simulink model "satellite_attitude_estimation_ekf_bst_model"  (R2017a)
settings: Solver=FixedStepAuto  StartTime=0.0  StopTime=10.0  FixedStep=dt  RelTol=1e-3
values from neighbouring files (symbols this model uses):
  ARW = N_ARW^2    (= 2.56183250041e-07)    [satellite_attitude_estimation_ekf_bst_run.m]
  dt = CONST.dt    [extended_kalman_filter.m]    (also in satellite_attitude_estimation_ekf_bst_run.m = 0.05)
  dt_mg = 1/20    (= 0.05)    [satellite_attitude_estimation_ekf_bst_run.m]
  dt_ss = 1/5    (= 0.2)    [satellite_attitude_estimation_ekf_bst_run.m]
  dt_st = 1    [satellite_attitude_estimation_ekf_bst_run.m]
  FOV = 70    [satellite_attitude_estimation_ekf_bst_run.m]
  Gg = eye(3).*(-0.01+0.02*rand(3))+              (ones(3,3)-eye(3)).*(-0.0006+0.0012*rand(3))    [satellite_attitude_estimation_ekf_bst_run.m]
  Gmg = eye(3).*(-0.02+0.04*rand(3)) +             (ones(3,3)-eye(3)).*(-0.0028+0.0056*rand(3))    [satellite_attitude_estimation_ekf_bst_run.m]
  GYRO_Bias = (3*randn(3,1))*pi/180    [satellite_attitude_estimation_ekf_bst_run.m]
  P = 2*pi*sqrt(a^3/CONST.mu)    [satellite_attitude_estimation_ekf_bst_run.m]
  q_B_I_0 = [q_I_B_0(1);-q_I_B_0(2);-q_I_B_0(3);-q_I_B_0(4)]    [satellite_attitude_estimation_ekf_bst_run.m]
  q_B_O_0 = [q_O_B_0(1);-q_O_B_0(2);-q_O_B_0(3);-q_O_B_0(4)]    [satellite_attitude_estimation_ekf_bst_run.m]
  R_S1_B = DCM(SSaxis(1),SSangles(1))    [satellite_attitude_estimation_ekf_bst_run.m]
  R_S2_B = DCM(SSaxis(2),SSangles(2))    [satellite_attitude_estimation_ekf_bst_run.m]
  R_S3_B = DCM(SSaxis(3),SSangles(3))    [satellite_attitude_estimation_ekf_bst_run.m]
  R_S4_B = DCM(SSaxis(4),SSangles(4))    [satellite_attitude_estimation_ekf_bst_run.m]
  RRW = K_RRW^2/3    (= 4.06156559716e-12)    [satellite_attitude_estimation_ekf_bst_run.m]
  sigMag = 1.25e-7    (= 1.25e-07)    [satellite_attitude_estimation_ekf_bst_run.m]
  sigSS = 0.1    [satellite_attitude_estimation_ekf_bst_run.m]
  varST = sigST^2    (= 1.27968566268e-08)    [satellite_attitude_estimation_ekf_bst_run.m]
  w_B_BI_0 = w_B_BO_0 + w_B_OI_0    [satellite_attitude_estimation_ekf_bst_run.m]
undefined symbols (not defined in the file or in its folder): R_0, V_0
libraries: simulink x5
settings Model: Creator=Rusty Goh  LastModifiedBy=Rusty Goh

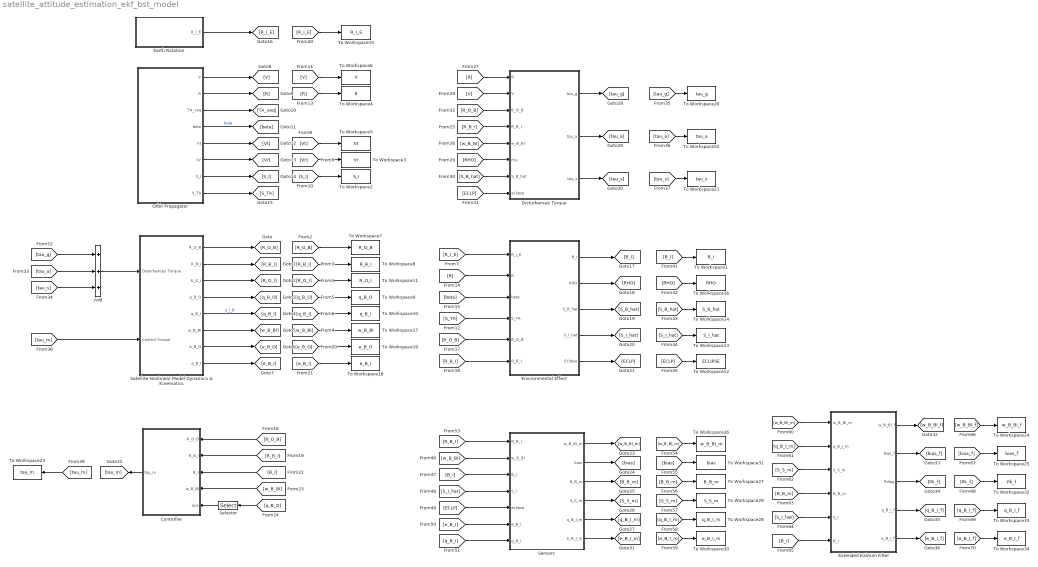
== system satellite_attitude_estimation_ekf_bst_model ==
  "\tOrbit Propagator" : Subsystem
  Add : Sum  Inputs=+++
  Controller : Subsystem
  Disturbances Torque : Subsystem
  Earth Rotation : Subsystem
  Environmental Effect : Subsystem
  Extended Kalman Filter : Subsystem
  Satellite Nonlinear Model Dynamics & Kinematics : Subsystem
  Selector : Selector  NumberOfDimensions=2  InputPortWidth=3  IndexOptions=Index vector (dialog),Index vector (dialog)  Indices=[2:4],1  OutputSizes=1,1
  Sensors : Subsystem
  To Workspace1 : ToWorkspace  VariableName=B_I  SampleTime=-1
  To Workspace10 : ToWorkspace  VariableName=q_B_I  SampleTime=-1
  To Workspace11 : ToWorkspace  VariableName=R_O_I  SampleTime=-1
  To Workspace12 : ToWorkspace  VariableName=ECLIPSE  SampleTime=-1
      settings: Save2DSignal=2-D array (concatenate along first dimension)
  To Workspace13 : ToWorkspace  VariableName=S_I_hat  SampleTime=-1
  To Workspace14 : ToWorkspace  VariableName=S_B_hat  SampleTime=-1
  To Workspace15 : ToWorkspace  VariableName=R_I_E  SampleTime=-1
  To Workspace16 : ToWorkspace  VariableName=RHO  SampleTime=-1
      settings: Save2DSignal=2-D array (concatenate along first dimension)
  To Workspace17 : ToWorkspace  VariableName=w_B_BI  SampleTime=-1
  To Workspace18 : ToWorkspace  VariableName=e_B_I  SampleTime=-1
  To Workspace19 : ToWorkspace  VariableName=e_B_O  SampleTime=-1
  To Workspace2 : ToWorkspace  VariableName=S_I  SampleTime=-1
  To Workspace20 : ToWorkspace  VariableName=tau_g  SampleTime=-1
  To Workspace21 : ToWorkspace  VariableName=tau_s  SampleTime=-1
  To Workspace22 : ToWorkspace  VariableName=tau_a  SampleTime=-1
      settings: Save2DSignal=2-D array (concatenate along first dimension)
  To Workspace23 : ToWorkspace  VariableName=tau_m  SampleTime=-1
  To Workspace24 : ToWorkspace  VariableName=w_B_BI_f  SampleTime=-1
  To Workspace25 : ToWorkspace  VariableName=bias_f  SampleTime=-1
  To Workspace26 : ToWorkspace  VariableName=w_B_BI_m  SampleTime=dt
  To Workspace27 : ToWorkspace  VariableName=B_B_m  SampleTime=dt
  To Workspace28 : ToWorkspace  VariableName=q_B_I_m  SampleTime=dt
  To Workspace29 : ToWorkspace  VariableName=S_S_m  SampleTime=dt
  To Workspace3 : ToWorkspace  VariableName=Vr  SampleTime=-1
  To Workspace30 : ToWorkspace  VariableName=e_B_I_m  SampleTime=dt
  To Workspace31 : ToWorkspace  VariableName=bias  SampleTime=dt
  To Workspace32 : ToWorkspace  VariableName=Pk_f  SampleTime=-1
  To Workspace33 : ToWorkspace  VariableName=q_B_I_f  SampleTime=-1
  To Workspace34 : ToWorkspace  VariableName=e_B_I_f  SampleTime=-1
  To Workspace4 : ToWorkspace  VariableName=R  SampleTime=-1
  To Workspace5 : ToWorkspace  VariableName=Vt  SampleTime=-1
  To Workspace6 : ToWorkspace  VariableName=V  SampleTime=-1
  To Workspace7 : ToWorkspace  VariableName=R_O_B  SampleTime=-1
  To Workspace8 : ToWorkspace  VariableName=R_B_I  SampleTime=-1
  To Workspace9 : ToWorkspace  VariableName=q_B_O  SampleTime=-1
  wires:
  Satellite Nonlinear Model Dynamics & Kinematics/4(q_B_O) -> [q_B_O]
  Satellite Nonlinear Model Dynamics & Kinematics/3(R_O_I) -> [R_O_I]
  Satellite Nonlinear Model Dynamics & Kinematics/1(R_O_B) -> [R_O_B]
  Satellite Nonlinear Model Dynamics & Kinematics/7(e_B_O) -> [e_B_O]
  Satellite Nonlinear Model Dynamics & Kinematics/5(q_B_I) -> [q_B_I]  "q_I_B"
  Satellite Nonlinear Model Dynamics & Kinematics/2(R_B_I) -> [R_B_I]
  Satellite Nonlinear Model Dynamics & Kinematics/6(w_B_BI) -> [w_B_BI]
  Satellite Nonlinear Model Dynamics & Kinematics/8(e_B_I) -> [e_B_I]
  Add/1 -> Satellite Nonlinear Model Dynamics & Kinematics/1(Disturbances Torque)
  "\tOrbit Propagator"/6(Vr) -> [Vr]
  "\tOrbit Propagator"/7("S_I ") -> [S_I]
  "\tOrbit Propagator"/3(TA_veq) -> [TA_veq]
  "\tOrbit Propagator"/4(beta) -> [beta]  "beta"
  "\tOrbit Propagator"/5(Vt) -> [Vt]
  "\tOrbit Propagator"/8(S_TA) -> [S_TA]
  "\tOrbit Propagator"/2(R) -> [R]
  "\tOrbit Propagator"/1(V) -> [V]
  [R] -> To Workspace4/1
  [Vr] -> To Workspace3/1
  [S_I] -> To Workspace2/1
  [Vt] -> To Workspace5/1
  [V] -> To Workspace6/1
  [R_O_B] -> To Workspace7/1
  [e_B_O] -> To Workspace19/1
  [w_B_BI] -> To Workspace17/1
  [R_O_I] -> To Workspace11/1
  [e_B_I] -> To Workspace18/1
  [R_B_I] -> To Workspace8/1
  [q_B_O] -> To Workspace9/1
  [q_B_I] -> To Workspace10/1
  [S_TA] -> Environmental Effect/4(S_TA)
  Environmental Effect/3(S_B_hat) -> [S_B_hat]
  [B_I] -> To Workspace1/1
  [ECLP] -> To Workspace12/1
  [R_I_E] -> To Workspace15/1
  [S_B_hat] -> To Workspace14/1
  [beta] -> Environmental Effect/3(beta)
  [R] -> Environmental Effect/2(R)
  Environmental Effect/5(Eclipse) -> [ECLP]
  [RHO] -> To Workspace16/1
  Environmental Effect/4(S_I_hat) -> [S_I_hat]
  Earth Rotation/1(R_I_E) -> [R_I_E]
  Environmental Effect/1(B_I) -> [B_I]
  Environmental Effect/2(RHO) -> [RHO]
  [S_I_hat] -> To Workspace13/1
  [R_B_I] -> Environmental Effect/6(R_B_I)
  [R_O_B] -> Environmental Effect/5(R_O_B)
  [R_I_E] -> Environmental Effect/1(R_I_E)
  Controller/1(tau_m) -> [tau_m]
  [R_O_B] -> Controller/1(R_O_B)
  [R_B_I] -> Controller/2(R_B_I)
  [B_I] -> Controller/3(B_I)
  [w_B_BI] -> Controller/4(w_B_BI)
  [q_B_O] -> Selector/1
  Selector/1 -> Controller/5(eps)
  [S_B_hat] -> Disturbances Torque/7(S_B_hat)
  [R_O_B] -> Disturbances Torque/3(R_O_B)
  [V] -> Disturbances Torque/2(V)
  Disturbances Torque/1(tau_g) -> [tau_g]
  [R_B_I] -> Disturbances Torque/4(R_B_I)
  [ECLP] -> Disturbances Torque/8(eclipse)
  [RHO] -> Disturbances Torque/6(rho)
  [w_B_BI] -> Disturbances Torque/5(w_B_BI)
  [R] -> Disturbances Torque/1(R)
  Disturbances Torque/2(tau_a) -> [tau_a]
  Disturbances Torque/3(tau_s) -> [tau_s]
  [tau_g] -> Add/1
  [tau_a] -> Add/2
  [tau_s] -> Add/3
  [tau_g] -> To Workspace20/1
  [tau_a] -> To Workspace22/1
  [tau_s] -> To Workspace21/1
  [tau_m] -> Satellite Nonlinear Model Dynamics & Kinematics/2(Control Torque)
  [tau_m] -> To Workspace23/1
  [S_S_m] -> To Workspace29/1
  [e_B_I_m] -> To Workspace30/1
  [B_B_m] -> To Workspace27/1
  [R_B_I] -> Sensors/1(R_B_I)
  [bias] -> To Workspace31/1
  [ECLP] -> Sensors/5(eclipse)
  [q_B_I] -> Sensors/7(q_B_I)
  [w_B_BI_m] -> To Workspace26/1
  [e_B_I] -> Sensors/6(e_B_I)
  Sensors/3(B_B_m) -> [B_B_m]
  Sensors/5(q_B_I_m) -> [q_B_I_m]
  [B_I] -> Sensors/3(B_I)
  Sensors/2(bias) -> [bias]
  Sensors/6(e_B_I_m) -> [e_B_I_m]
  [w_B_BI] -> Sensors/2(w_B_BI)
  [S_I_hat] -> Sensors/4(S_I)
  Sensors/4(S_S_m) -> [S_S_m]
  Sensors/1(w_B_BI_m) -> [w_B_BI_m]
  [q_B_I_m] -> To Workspace28/1
  [S_S_m] -> Extended Kalman Filter/3(S_S_m)
  Extended Kalman Filter/3(Pdiag) -> [Pk_f]
  Extended Kalman Filter/2(bias_f) -> [bias_f]
  [e_B_I_f] -> To Workspace34/1
  Extended Kalman Filter/4(q_B_I_f) -> [q_B_I_f]
  [Pk_f] -> To Workspace32/1
  [bias_f] -> To Workspace25/1
  [B_B_m] -> Extended Kalman Filter/4(B_B_m)
  [q_B_I_m] -> Extended Kalman Filter/2(q_B_I_m)
  Extended Kalman Filter/1(w_B_BI_f) -> [w_B_BI_f]
  [w_B_BI_f] -> To Workspace24/1
  [S_I_hat] -> Extended Kalman Filter/5(S_I)
  [q_B_I_f] -> To Workspace33/1
  [B_I] -> Extended Kalman Filter/6(B_I)
  Extended Kalman Filter/5(e_B_I_f) -> [e_B_I_f]
  [w_B_BI_m] -> Extended Kalman Filter/1(w_B_BI_m)

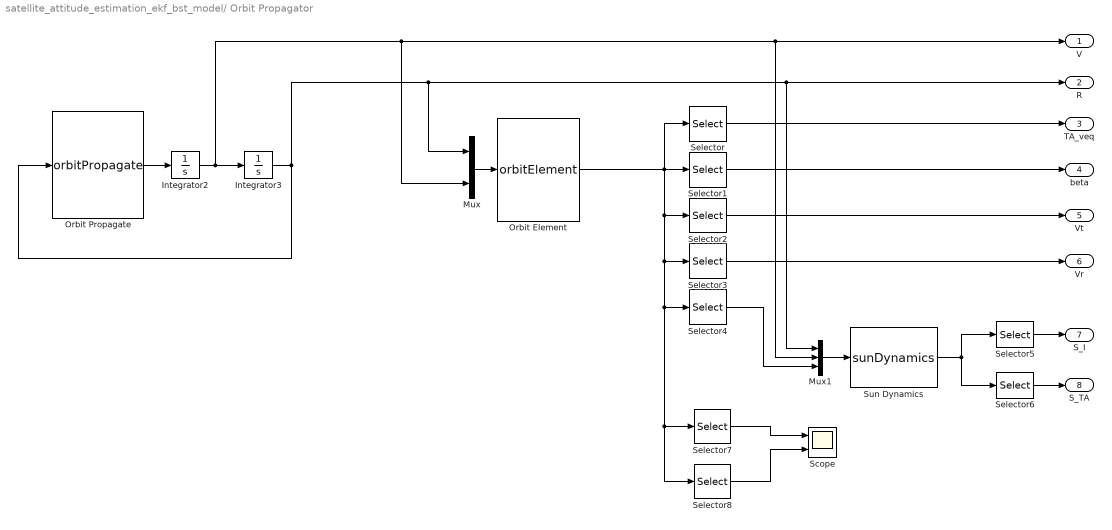
== system satellite_attitude_estimation_ekf_bst_model/	Orbit Propagator ==
  Integrator2 : Integrator  InitialCondition=V_0
  Integrator3 : Integrator  InitialCondition=R_0
  Mux : Mux  Inputs=2
  Mux1 : Mux  Inputs=3
  Orbit Element : MATLABFcn  MATLABFcn=orbitElement  OutputDimensions=11  Output1D=off
  Orbit Propagate : MATLABFcn  MATLABFcn=orbitPropagate  OutputDimensions=[3,1]  Output1D=off
  Scope : Scope  NumInputPorts=2
  Selector : Selector  InputPortWidth=11  IndexOptions=Index vector (dialog)  Indices=1  OutputSizes=1
  Selector1 : Selector  InputPortWidth=11  IndexOptions=Index vector (dialog)  Indices=2  OutputSizes=1
  Selector2 : Selector  InputPortWidth=11  IndexOptions=Index vector (dialog)  Indices=[3:5]  OutputSizes=1
  Selector3 : Selector  InputPortWidth=11  IndexOptions=Index vector (dialog)  Indices=[6:8]  OutputSizes=1
  Selector4 : Selector  InputPortWidth=11  IndexOptions=Index vector (dialog)  Indices=9  OutputSizes=1
  Selector5 : Selector  NumberOfDimensions=2  InputPortWidth=4  IndexOptions=Index vector (dialog),Index vector (dialog)  Indices=1:3,1  OutputSizes=1,1
  Selector6 : Selector  NumberOfDimensions=2  InputPortWidth=4  IndexOptions=Index vector (dialog),Index vector (dialog)  Indices=4,1  OutputSizes=1,1
  Selector7 : Selector  InputPortWidth=11  IndexOptions=Index vector (dialog)  Indices=10  OutputSizes=1
  Selector8 : Selector  InputPortWidth=11  IndexOptions=Index vector (dialog)  Indices=11  OutputSizes=1
  Sun Dynamics : MATLABFcn  MATLABFcn=sunDynamics  OutputDimensions=[4,1]  Output1D=off
  V : Outport
  R : Outport  Port=2
  TA_veq : Outport  Port=3
  beta : Outport  Port=4
  Vt : Outport  Port=5
  Vr : Outport  Port=6
  "S_I " : Outport  Port=7
  S_TA : Outport  Port=8
  wires:
  Mux/1 -> Orbit Element/1
  Orbit Element/1 -> Selector/1, Selector8/1, Selector7/1, Selector4/1, Selector3/1, Selector2/1, Selector1/1
  Orbit Propagate/1 -> Integrator2/1
  Integrator3/1 -> Mux/1, R/1, Mux1/1, Orbit Propagate/1
  Integrator2/1 -> Mux/2, Mux1/2, V/1, Integrator3/1
  Selector3/1 -> Vr/1
  Selector/1 -> TA_veq/1
  Selector2/1 -> Vt/1
  Selector1/1 -> beta/1
  Sun Dynamics/1 -> Selector6/1, Selector5/1
  Selector4/1 -> Mux1/3
  Selector6/1 -> S_TA/1
  Selector5/1 -> "S_I "/1
  Mux1/1 -> Sun Dynamics/1
  Selector7/1 -> Scope/1
  Selector8/1 -> Scope/2

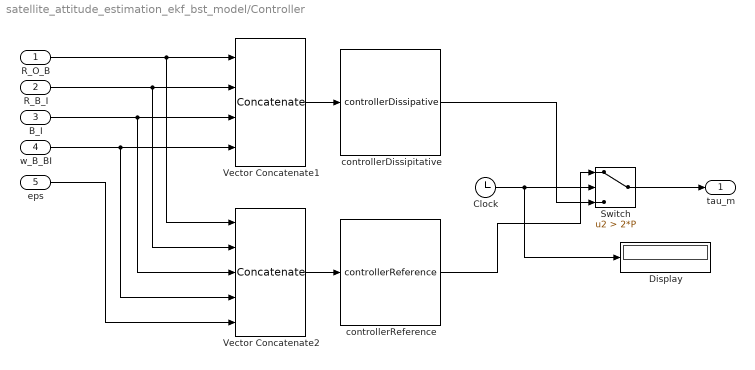
== system satellite_attitude_estimation_ekf_bst_model/Controller ==
  R_O_B : Inport
  R_B_I : Inport  Port=2
  B_I : Inport  Port=3
  w_B_BI : Inport  Port=4
  eps : Inport  Port=5
  Clock : Clock
  Display : Display
  Switch : Switch  Criteria=u2 > Threshold  Threshold=2*P
  Vector Concatenate1 : Concatenate  NumInputs=4  Mode=Multidimensional array  ConcatenateDimension=2
  Vector Concatenate2 : Concatenate  NumInputs=5  Mode=Multidimensional array  ConcatenateDimension=2
  controllerDissipitative : MATLABFcn  MATLABFcn=controllerDissipative  OutputDimensions=[3,1]  Output1D=off
  controllerReference : MATLABFcn  MATLABFcn=controllerReference  OutputDimensions=[3,1]  Output1D=off
  tau_m : Outport
  wires:
  Vector Concatenate1/1 -> controllerDissipitative/1
  R_O_B/1 -> Vector Concatenate2/1, Vector Concatenate1/1
  controllerDissipitative/1 -> Switch/3
  R_B_I/1 -> Vector Concatenate2/2, Vector Concatenate1/2
  B_I/1 -> Vector Concatenate2/3, Vector Concatenate1/3
  w_B_BI/1 -> Vector Concatenate2/4, Vector Concatenate1/4
  Vector Concatenate2/1 -> controllerReference/1
  eps/1 -> Vector Concatenate2/5
  controllerReference/1 -> Switch/1
  Clock/1 -> Display/1, Switch/2
  Switch/1 -> tau_m/1

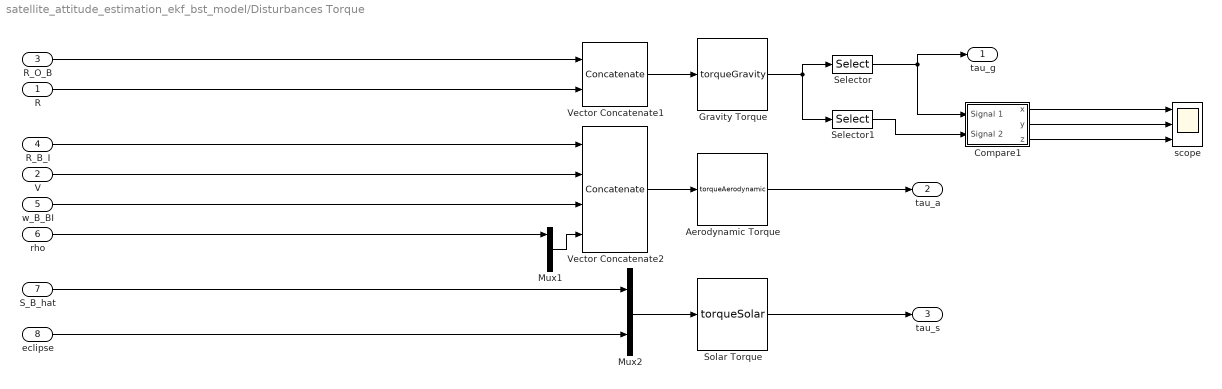
== system satellite_attitude_estimation_ekf_bst_model/Disturbances Torque ==
  R : Inport
  V : Inport  Port=2
  R_O_B : Inport  Port=3
  R_B_I : Inport  Port=4
  w_B_BI : Inport  Port=5
  rho : Inport  Port=6
  S_B_hat : Inport  Port=7
  eclipse : Inport  Port=8
  Aerodynamic Torque : MATLABFcn  MATLABFcn=torqueAerodynamic  OutputDimensions=[3,1]  Output1D=off
  Compare1 : Subsystem
  Gravity Torque : MATLABFcn  MATLABFcn=torqueGravity  OutputDimensions=[3,2]  Output1D=off
  Mux1 : Mux  Inputs=3
  Mux2 : Mux  Inputs=2
  Selector : Selector  NumberOfDimensions=2  InputPortWidth=3  IndexOptions=Index vector (dialog),Index vector (dialog)  Indices=[1:3],1  OutputSizes=1,1
  Selector1 : Selector  NumberOfDimensions=2  InputPortWidth=3  IndexOptions=Index vector (dialog),Index vector (dialog)  Indices=[1:3],2  OutputSizes=1,1
  Solar Torque : MATLABFcn  MATLABFcn=torqueSolar  OutputDimensions=[3,1]  Output1D=off
  Vector Concatenate1 : Concatenate  Mode=Multidimensional array  ConcatenateDimension=2
  Vector Concatenate2 : Concatenate  NumInputs=4  Mode=Multidimensional array  ConcatenateDimension=2
  scope : Scope  NumInputPorts=3
  tau_g : Outport
  tau_a : Outport  Port=2
  tau_s : Outport  Port=3
  wires:
  Vector Concatenate2/1 -> Aerodynamic Torque/1
  Mux1/1 -> Vector Concatenate2/4
  Vector Concatenate1/1 -> Gravity Torque/1
  Mux2/1 -> Solar Torque/1
  S_B_hat/1 -> Mux2/1
  w_B_BI/1 -> Vector Concatenate2/3
  R_B_I/1 -> Vector Concatenate2/1
  V/1 -> Vector Concatenate2/2
  R/1 -> Vector Concatenate1/2
  R_O_B/1 -> Vector Concatenate1/1
  rho/1 -> Mux1/1
  eclipse/1 -> Mux2/2
  Gravity Torque/1 -> Selector1/1, Selector/1
  Aerodynamic Torque/1 -> tau_a/1
  Solar Torque/1 -> tau_s/1
  Selector/1 -> tau_g/1, Compare1/1(Signal 1)
  Compare1/1(x) -> scope/1
  Compare1/2(y) -> scope/2
  Compare1/3(z) -> scope/3
  Selector1/1 -> Compare1/2(Signal 2)

== system satellite_attitude_estimation_ekf_bst_model/Earth Rotation ==
  Clock : Clock
  Interpreted MATLAB Function : MATLABFcn  MATLABFcn=earthDynamics  OutputDimensions=[3,3]  Output1D=off
  R_I_E : Outport
  wires:
  Interpreted MATLAB Function/1 -> R_I_E/1
  Clock/1 -> Interpreted MATLAB Function/1

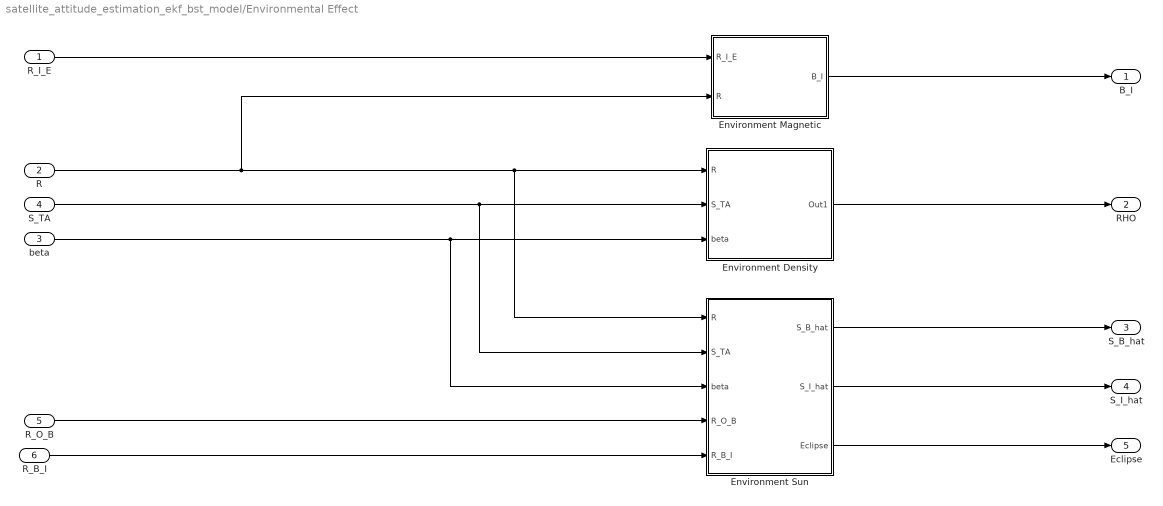
== system satellite_attitude_estimation_ekf_bst_model/Environmental Effect ==
  R_I_E : Inport
  R : Inport  Port=2
  beta : Inport  Port=3
  S_TA : Inport  Port=4
  R_O_B : Inport  Port=5
  R_B_I : Inport  Port=6
  Environment Density : Subsystem
  Environment Magnetic : Subsystem
  Environment Sun : Subsystem
  B_I : Outport
  RHO : Outport  Port=2
  S_B_hat : Outport  Port=3
  S_I_hat : Outport  Port=4
  Eclipse : Outport  Port=5
  wires:
  S_TA/1 -> Environment Sun/2(S_TA), Environment Density/2(S_TA)
  beta/1 -> Environment Sun/3(beta), Environment Density/3(beta)
  R_O_B/1 -> Environment Sun/4(R_O_B)
  R_B_I/1 -> Environment Sun/5(R_B_I)
  Environment Sun/1(S_B_hat) -> S_B_hat/1
  Environment Sun/2(S_I_hat) -> S_I_hat/1
  Environment Sun/3(Eclipse) -> Eclipse/1
  R/1 -> Environment Magnetic/2(R), Environment Sun/1(R), Environment Density/1(R)
  Environment Density/1(Out1) -> RHO/1
  R_I_E/1 -> Environment Magnetic/1(R_I_E)
  Environment Magnetic/1(B_I) -> B_I/1

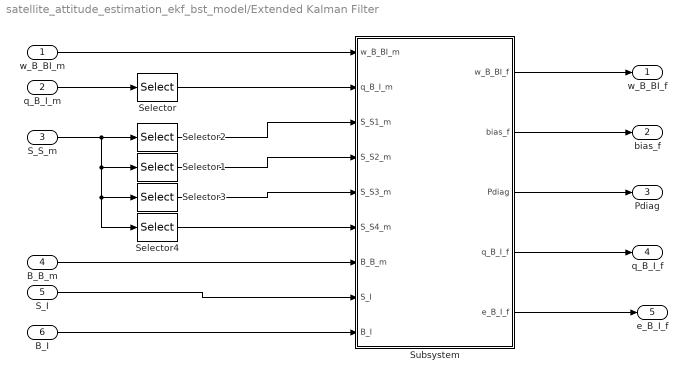
== system satellite_attitude_estimation_ekf_bst_model/Extended Kalman Filter ==
  w_B_BI_m : Inport
  q_B_I_m : Inport  Port=2
  S_S_m : Inport  Port=3
  B_B_m : Inport  Port=4
  S_I : Inport  Port=5
  B_I : Inport  Port=6
  Selector : Selector  InputPortWidth=4  IndexOptions=Index vector (dialog)  Indices=[2:4]  OutputSizes=1
  Selector1 : Selector  NumberOfDimensions=2  InputPortWidth=4  IndexOptions=Index vector (dialog),Index vector (dialog)  Indices=[1:3],2  OutputSizes=1,1
  Selector2 : Selector  NumberOfDimensions=2  InputPortWidth=4  IndexOptions=Index vector (dialog),Index vector (dialog)  Indices=[1:3],1  OutputSizes=1,1
  Selector3 : Selector  NumberOfDimensions=2  InputPortWidth=4  IndexOptions=Index vector (dialog),Index vector (dialog)  Indices=[1:3],3  OutputSizes=1,1
  Selector4 : Selector  NumberOfDimensions=2  InputPortWidth=4  IndexOptions=Index vector (dialog),Index vector (dialog)  Indices=[1:3],4  OutputSizes=1,1
  Subsystem : Subsystem
  w_B_BI_f : Outport
  bias_f : Outport  Port=2
  Pdiag : Outport  Port=3
  q_B_I_f : Outport  Port=4
  e_B_I_f : Outport  Port=5
  wires:
  q_B_I_m/1 -> Selector/1
  w_B_BI_m/1 -> Subsystem/1(w_B_BI_m)
  Selector2/1 -> Subsystem/3(S_S1_m)
  Selector1/1 -> Subsystem/4(S_S2_m)
  B_B_m/1 -> Subsystem/7(B_B_m)
  B_I/1 -> Subsystem/9(B_I)
  Selector/1 -> Subsystem/2(q_B_I_m)
  S_I/1 -> Subsystem/8(S_I)
  Subsystem/1(w_B_BI_f) -> w_B_BI_f/1
  Subsystem/2(bias_f) -> bias_f/1
  Subsystem/3(Pdiag) -> Pdiag/1
  Subsystem/4(q_B_I_f) -> q_B_I_f/1
  Subsystem/5(e_B_I_f) -> e_B_I_f/1
  S_S_m/1 -> Selector2/1, Selector4/1, Selector3/1, Selector1/1
  Selector3/1 -> Subsystem/5(S_S3_m)
  Selector4/1 -> Subsystem/6(S_S4_m)

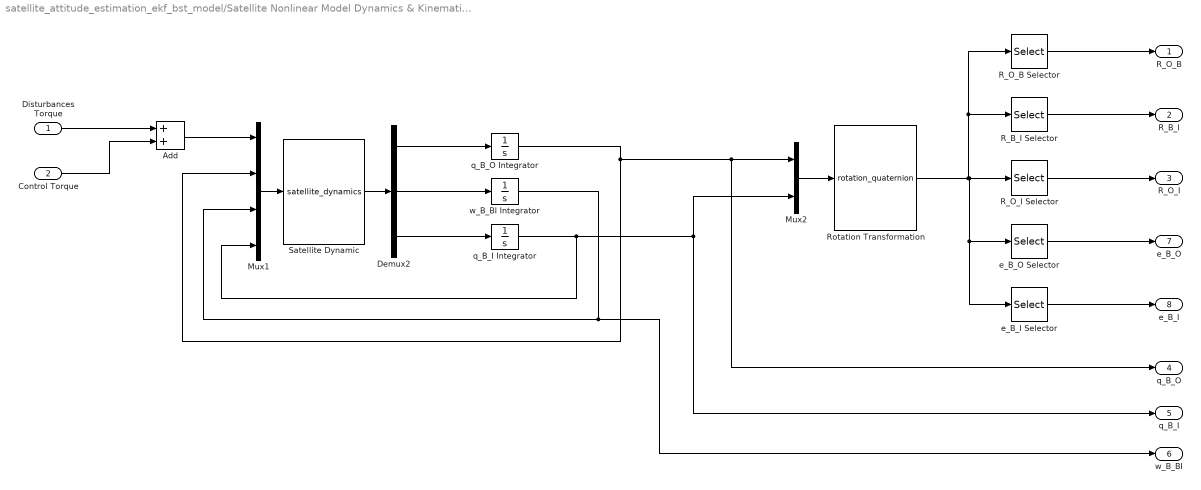
== system satellite_attitude_estimation_ekf_bst_model/Satellite Nonlinear Model Dynamics & Kinematics ==
  Disturbances Torque : Inport
  Control Torque : Inport  Port=2
  " w_B_BI Integrator" : Integrator  InitialCondition=w_B_BI_0
  Add : Sum
  Demux2 : Demux  Outputs=[4 3 4]
  Mux1 : Mux  Inputs=[3 4 3 4]
  Mux2 : Mux  Inputs=[4 4]
  R_B_I Selector : Selector  NumberOfDimensions=2  InputPortWidth=3  IndexOptions=Index vector (dialog),Index vector (dialog)  Indices=[1:3],[4:6]  OutputSizes=1,1
  R_O_B Selector : Selector  NumberOfDimensions=2  InputPortWidth=3  IndexOptions=Index vector (dialog),Index vector (dialog)  Indices=[1:3],[1:3]  OutputSizes=1,1
  R_O_I Selector : Selector  NumberOfDimensions=2  InputPortWidth=3  IndexOptions=Index vector (dialog),Index vector (dialog)  Indices=[1:3],[7:9]  OutputSizes=1,1
  Rotation Transformation : MATLABFcn  MATLABFcn=rotation_quaternion  OutputDimensions=[3,11]  Output1D=off
  Satellite Dynamic : MATLABFcn  MATLABFcn=satellite_dynamics  OutputDimensions=[11,1]  Output1D=off
  e_B_I Selector : Selector  NumberOfDimensions=2  InputPortWidth=3  IndexOptions=Index vector (dialog),Index vector (dialog)  Indices=[1:3],11  OutputSizes=1,1
  e_B_O Selector : Selector  NumberOfDimensions=2  InputPortWidth=3  IndexOptions=Index vector (dialog),Index vector (dialog)  Indices=[1:3],10  OutputSizes=1,1
  q_B_I Integrator : Integrator  InitialCondition=q_B_I_0
  q_B_O Integrator : Integrator  InitialCondition=q_B_O_0
  R_O_B : Outport
  R_B_I : Outport  Port=2
  R_O_I : Outport  Port=3
  q_B_O : Outport  Port=4
  q_B_I : Outport  Port=5
  w_B_BI : Outport  Port=6
  e_B_O : Outport  Port=7
  e_B_I : Outport  Port=8
  wires:
  R_O_I Selector/1 -> R_O_I/1
  q_B_O Integrator/1 -> Mux2/1, q_B_O/1, Mux1/2
  Satellite Dynamic/1 -> Demux2/1
  Disturbances Torque/1 -> Add/1
  Demux2/2 -> " w_B_BI Integrator"/1
  Demux2/3 -> q_B_I Integrator/1
  q_B_I Integrator/1 -> Mux2/2, q_B_I/1, Mux1/4
  Mux1/1 -> Satellite Dynamic/1
  Rotation Transformation/1 -> R_O_B Selector/1, R_B_I Selector/1, e_B_I Selector/1, e_B_O Selector/1, R_O_I Selector/1
  " w_B_BI Integrator"/1 -> w_B_BI/1, Mux1/3
  Demux2/1 -> q_B_O Integrator/1
  Mux2/1 -> Rotation Transformation/1
  R_B_I Selector/1 -> R_B_I/1
  R_O_B Selector/1 -> R_O_B/1
  Control Torque/1 -> Add/2
  Add/1 -> Mux1/1
  e_B_I Selector/1 -> e_B_I/1
  e_B_O Selector/1 -> e_B_O/1

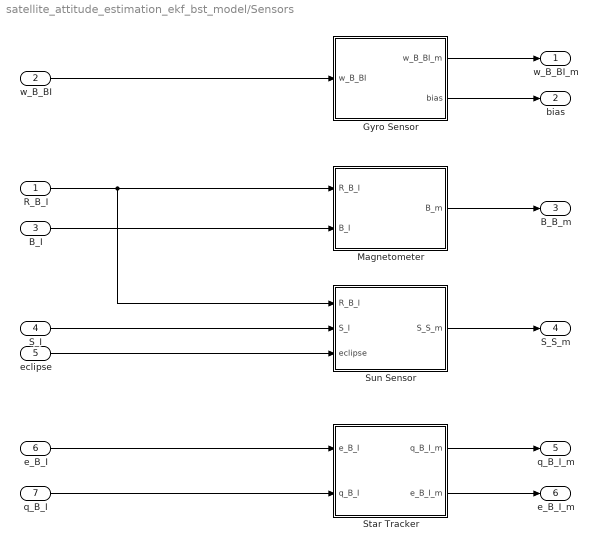
== system satellite_attitude_estimation_ekf_bst_model/Sensors ==
  R_B_I : Inport
  w_B_BI : Inport  Port=2
  B_I : Inport  Port=3
  S_I : Inport  Port=4
  eclipse : Inport  Port=5
  e_B_I : Inport  Port=6
  q_B_I : Inport  Port=7
  Gyro Sensor : Subsystem
  Magnetometer : Subsystem
  Star Tracker : Subsystem
  Sun Sensor : Subsystem
  w_B_BI_m : Outport
  bias : Outport  Port=2
  B_B_m : Outport  Port=3
  S_S_m : Outport  Port=4
  q_B_I_m : Outport  Port=5
  e_B_I_m : Outport  Port=6
  wires:
  e_B_I/1 -> Star Tracker/1(e_B_I)
  B_I/1 -> Magnetometer/2(B_I)
  eclipse/1 -> Sun Sensor/3(eclipse)
  Sun Sensor/1(S_S_m) -> S_S_m/1
  Gyro Sensor/2(bias) -> bias/1
  Gyro Sensor/1(w_B_BI_m) -> w_B_BI_m/1
  Star Tracker/1(q_B_I_m) -> q_B_I_m/1
  Magnetometer/1(B_m) -> B_B_m/1
  w_B_BI/1 -> Gyro Sensor/1(w_B_BI)
  S_I/1 -> Sun Sensor/2(S_I)
  R_B_I/1 -> Sun Sensor/1(R_B_I), Magnetometer/1(R_B_I)
  q_B_I/1 -> Star Tracker/2(q_B_I)
  Star Tracker/2(e_B_I_m) -> e_B_I_m/1

== system satellite_attitude_estimation_ekf_bst_model/Disturbances Torque/Compare1 ==
  Signal 1 : Inport
  Signal 2 : Inport  Port=2
  Demux3 : Demux  Outputs=3
  Demux4 : Demux  Outputs=3
  Mux : Mux  Inputs=2
  Mux1 : Mux  Inputs=2
  Mux2 : Mux  Inputs=2
  x : Outport
  y : Outport  Port=2
  z : Outport  Port=3
  wires:
  Demux3/3 -> Mux2/2
  Demux3/2 -> Mux1/2
  Demux4/2 -> Mux1/1
  Demux3/1 -> Mux/2
  Mux/1 -> x/1
  Mux2/1 -> z/1
  Demux4/1 -> Mux/1
  Mux1/1 -> y/1
  Demux4/3 -> Mux2/1
  Signal 2/1 -> Demux3/1
  Signal 1/1 -> Demux4/1

== system satellite_attitude_estimation_ekf_bst_model/Environmental Effect/Environment Density ==
  R : Inport
  S_TA : Inport  Port=2
  beta : Inport  Port=3
  Environment Density : MATLABFcn  MATLABFcn=environmentDensity  OutputDimensions=1  Output1D=off
  Mux : Mux  Inputs=3
  Out1 : Outport
  wires:
  Mux/1 -> Environment Density/1
  Environment Density/1 -> Out1/1
  S_TA/1 -> Mux/2
  beta/1 -> Mux/3
  R/1 -> Mux/1

== system satellite_attitude_estimation_ekf_bst_model/Environmental Effect/Environment Magnetic ==
  R_I_E : Inport
  R : Inport  Port=2
  Environment Magnetic : MATLABFcn  MATLABFcn=environmentMagnetic  OutputDimensions=[3,1]  Output1D=off
  Vector Concatenate : Concatenate  Mode=Multidimensional array  ConcatenateDimension=2
  B_I : Outport
  wires:
  R_I_E/1 -> Vector Concatenate/1
  Vector Concatenate/1 -> Environment Magnetic/1
  R/1 -> Vector Concatenate/2
  Environment Magnetic/1 -> B_I/1

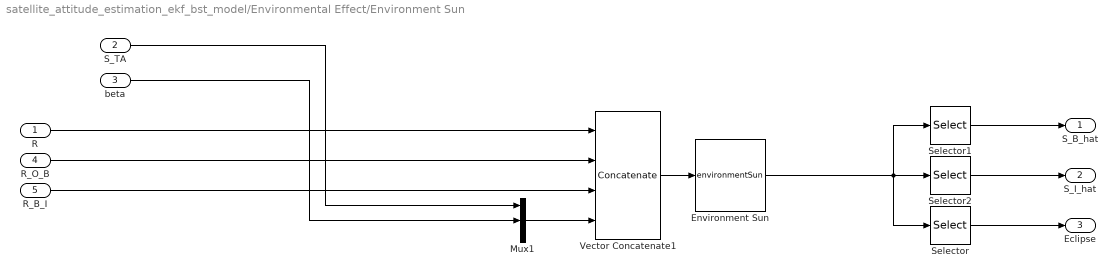
== system satellite_attitude_estimation_ekf_bst_model/Environmental Effect/Environment Sun ==
  R : Inport
  S_TA : Inport  Port=2
  beta : Inport  Port=3
  R_O_B : Inport  Port=4
  R_B_I : Inport  Port=5
  Environment Sun : MATLABFcn  MATLABFcn=environmentSun  OutputDimensions=[3,3]  Output1D=off
  Mux1 : Mux  Inputs=3
  Selector : Selector  NumberOfDimensions=2  InputPortWidth=3  IndexOptions=Index vector (dialog),Index vector (dialog)  Indices=3,3  OutputSizes=1,1
  Selector1 : Selector  NumberOfDimensions=2  InputPortWidth=3  IndexOptions=Index vector (dialog),Index vector (dialog)  Indices=[1:3],1  OutputSizes=1,1
  Selector2 : Selector  NumberOfDimensions=2  InputPortWidth=3  IndexOptions=Index vector (dialog),Index vector (dialog)  Indices=[1:3],2  OutputSizes=1,1
  Vector Concatenate1 : Concatenate  NumInputs=4  Mode=Multidimensional array  ConcatenateDimension=2
  S_B_hat : Outport
  S_I_hat : Outport  Port=2
  Eclipse : Outport  Port=3
  wires:
  R/1 -> Vector Concatenate1/1
  Mux1/1 -> Vector Concatenate1/4
  Selector/1 -> Eclipse/1
  Selector1/1 -> S_B_hat/1
  Vector Concatenate1/1 -> Environment Sun/1
  R_O_B/1 -> Vector Concatenate1/2
  R_B_I/1 -> Vector Concatenate1/3
  Selector2/1 -> S_I_hat/1
  Environment Sun/1 -> Selector/1, Selector1/1, Selector2/1
  S_TA/1 -> Mux1/1
  beta/1 -> Mux1/2

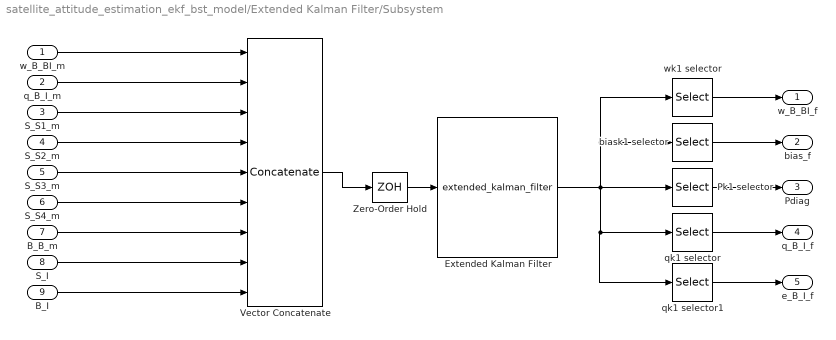
== system satellite_attitude_estimation_ekf_bst_model/Extended Kalman Filter/Subsystem ==
  w_B_BI_m : Inport
  q_B_I_m : Inport  Port=2
  S_S1_m : Inport  Port=3
  S_S2_m : Inport  Port=4
  S_S3_m : Inport  Port=5
  S_S4_m : Inport  Port=6
  B_B_m : Inport  Port=7
  S_I : Inport  Port=8
  B_I : Inport  Port=9
  Extended Kalman Filter : MATLABFcn  MATLABFcn=extended_kalman_filter  OutputDimensions=[6,9]  Output1D=off
  Pk1 selector : Selector  NumberOfDimensions=2  InputPortWidth=3  IndexOptions=Index vector (dialog),Index vector (dialog)  Indices=[1:6],[2:7]  OutputSizes=1,1
  Vector Concatenate : Concatenate  NumInputs=9  Mode=Multidimensional array  ConcatenateDimension=2
  Zero-Order Hold : ZeroOrderHold  SampleTime=dt
  biask1 selector : Selector  NumberOfDimensions=2  InputPortWidth=3  IndexOptions=Index vector (dialog),Index vector (dialog)  Indices=[4:6],1  OutputSizes=1,1
  qk1 selector : Selector  NumberOfDimensions=2  InputPortWidth=3  IndexOptions=Index vector (dialog),Index vector (dialog)  Indices=[1:4],8  OutputSizes=1,1
  qk1 selector1 : Selector  NumberOfDimensions=2  InputPortWidth=3  IndexOptions=Index vector (dialog),Index vector (dialog)  Indices=[1:3],9  OutputSizes=1,1
  wk1 selector : Selector  NumberOfDimensions=2  InputPortWidth=3  IndexOptions=Index vector (dialog),Index vector (dialog)  Indices=[1:3],1  OutputSizes=1,1
  w_B_BI_f : Outport
  bias_f : Outport  Port=2
  Pdiag : Outport  Port=3
  q_B_I_f : Outport  Port=4
  e_B_I_f : Outport  Port=5
  wires:
  Vector Concatenate/1 -> Zero-Order Hold/1
  S_S2_m/1 -> Vector Concatenate/4
  Pk1 selector/1 -> Pdiag/1
  qk1 selector1/1 -> e_B_I_f/1
  qk1 selector/1 -> q_B_I_f/1
  B_B_m/1 -> Vector Concatenate/7
  S_S1_m/1 -> Vector Concatenate/3
  Extended Kalman Filter/1 -> wk1 selector/1, biask1 selector/1, qk1 selector1/1, qk1 selector/1, Pk1 selector/1
  S_I/1 -> Vector Concatenate/8
  q_B_I_m/1 -> Vector Concatenate/2
  wk1 selector/1 -> w_B_BI_f/1
  w_B_BI_m/1 -> Vector Concatenate/1
  B_I/1 -> Vector Concatenate/9
  biask1 selector/1 -> bias_f/1
  Zero-Order Hold/1 -> Extended Kalman Filter/1
  S_S3_m/1 -> Vector Concatenate/5
  S_S4_m/1 -> Vector Concatenate/6

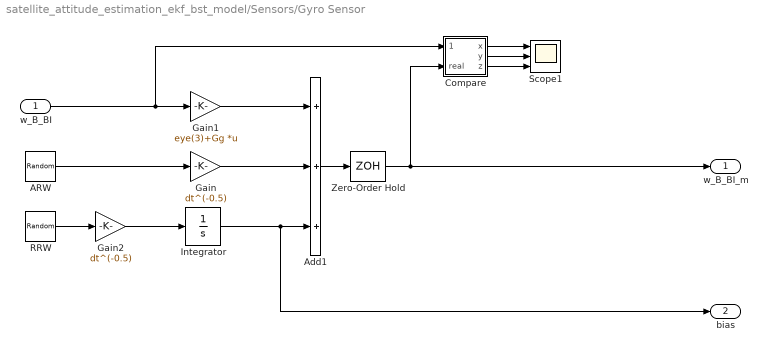
== system satellite_attitude_estimation_ekf_bst_model/Sensors/Gyro Sensor ==
  w_B_BI : Inport
  ARW : RandomNumber  Variance=[ARW;ARW;ARW]  SampleTime=dt  VectorParams1D=off
  Add1 : Sum  Inputs=+++
  Compare : Subsystem
  Gain : Gain  Gain=dt^(-0.5)
  Gain1 : Gain  Gain=eye(3)+Gg  Multiplication=Matrix(K*u)
  Gain2 : Gain  Gain=dt^(-0.5)
  Integrator : Integrator  InitialCondition=GYRO_Bias
  RRW : RandomNumber  Variance=[RRW;RRW;RRW]  SampleTime=dt  VectorParams1D=off
  Scope1 : Scope  NumInputPorts=3
  Zero-Order Hold : ZeroOrderHold  SampleTime=dt
  w_B_BI_m : Outport
  bias : Outport  Port=2
  wires:
  w_B_BI/1 -> Compare/1(true), Gain1/1
  Gain/1 -> Add1/2
  ARW/1 -> Gain/1
  Add1/1 -> Zero-Order Hold/1
  RRW/1 -> Gain2/1
  Integrator/1 -> Add1/3, bias/1
  Gain1/1 -> Add1/1
  Zero-Order Hold/1 -> w_B_BI_m/1, Compare/2(real)
  Compare/2(y) -> Scope1/2
  Compare/3(z) -> Scope1/3
  Compare/1(x) -> Scope1/1
  Gain2/1 -> Integrator/1

== system satellite_attitude_estimation_ekf_bst_model/Sensors/Magnetometer ==
  R_B_I : Inport
  B_I : Inport  Port=2
  ARW : RandomNumber  Variance=[sigMag^2;sigMag^2;sigMag^2]  SampleTime=dt_mg  VectorParams1D=off
  Add1 : Sum
  Compare : Subsystem
  Matrix Multiply : Product  Multiplication=Matrix(*)
  ScaleFactor MissAlignment : Gain  Gain=eye(3) + Gmg  Multiplication=Matrix(K*u)
  Scope1 : Scope  NumInputPorts=3
  Zero-Order Hold : ZeroOrderHold  SampleTime=dt_mg
  B_m : Outport
  wires:
  Matrix Multiply/1 -> Compare/1(true), ScaleFactor MissAlignment/1  "B_B"
  ScaleFactor MissAlignment/1 -> Add1/1
  Add1/1 -> Zero-Order Hold/1
  ARW/1 -> Add1/2
  B_I/1 -> Matrix Multiply/2
  R_B_I/1 -> Matrix Multiply/1
  Compare/2(y) -> Scope1/2
  Compare/3(z) -> Scope1/3
  Compare/1(x) -> Scope1/1
  Zero-Order Hold/1 -> Compare/2(real), B_m/1

== system satellite_attitude_estimation_ekf_bst_model/Sensors/Star Tracker ==
  e_B_I : Inport
  q_B_I : Inport  Port=2
  Mux : Mux  Inputs=2
  ST Noise : RandomNumber  Variance=[varST;varST;varST]  SampleTime=dt_st  VectorParams1D=off
  Selector : Selector  InputPortWidth=8  IndexOptions=Index vector (dialog)  Indices=[1:4]  OutputSizes=1
  Star Tracker : MATLABFcn  MATLABFcn=sensor_startracker  OutputDimensions=[8,1]  Output1D=off
  Sum : Sum  Inputs=|++
  Zero-Order Hold : ZeroOrderHold  SampleTime=dt_st
  q_B_I_m : Outport
  e_B_I_m : Outport  Port=2
  wires:
  Mux/1 -> Star Tracker/1
  Selector/1 -> Zero-Order Hold/1
  ST Noise/1 -> Sum/2
  e_B_I/1 -> Sum/1
  Star Tracker/1 -> Selector/1
  Zero-Order Hold/1 -> q_B_I_m/1
  Sum/1 -> e_B_I_m/1, Mux/2
  q_B_I/1 -> Mux/1

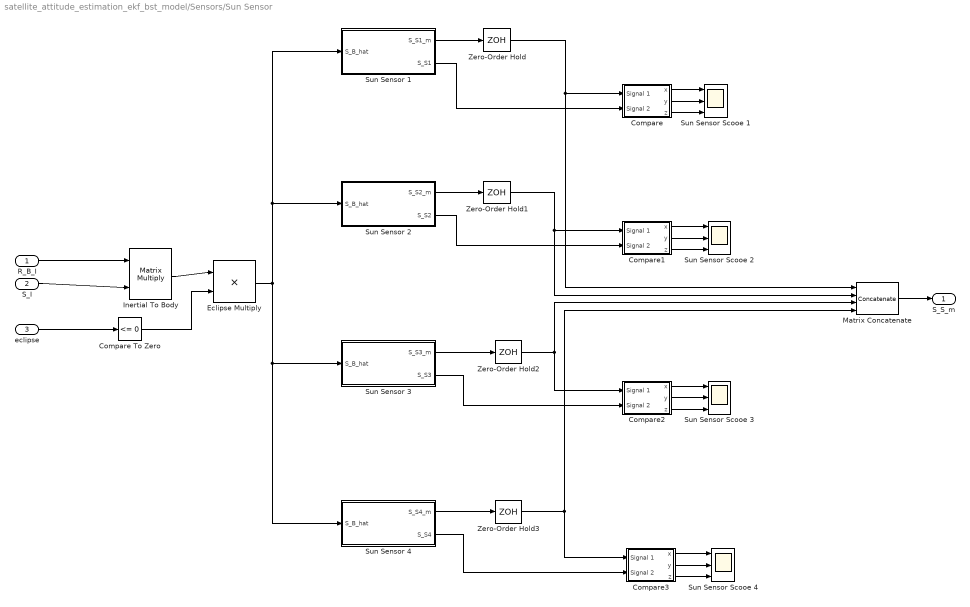
== system satellite_attitude_estimation_ekf_bst_model/Sensors/Sun Sensor ==
  R_B_I : Inport
  S_I : Inport  Port=2
  eclipse : Inport  Port=3
  Compare : Subsystem
  Compare To Zero : simulink/Logic and Bit Operations/Compare To Zero  relop=<=  OutDataTypeStr=boolean
  Compare1 : Subsystem
  Compare2 : Subsystem
  Compare3 : Subsystem
  Eclipse Multiply : Product
  Inertial To Body : Product  Multiplication=Matrix(*)
  Matrix Concatenate : Concatenate  NumInputs=4  Mode=Multidimensional array  ConcatenateDimension=2
  Sun Sensor Scooe {1..4} (4 alike) : Scope  NumInputPorts=3
  Sun Sensor 1 : Subsystem
  Sun Sensor 2 : Subsystem
  Sun Sensor 3 : Subsystem
  Sun Sensor 4 : Subsystem
  Zero-Order Hold{,1..3} (4 alike) : ZeroOrderHold  SampleTime=dt_ss
  S_S_m : Outport
  wires:
  R_B_I/1 -> Inertial To Body/1
  S_I/1 -> Inertial To Body/2
  Eclipse Multiply/1 -> Sun Sensor 1/1(S_B_hat), Sun Sensor 2/1(S_B_hat), Sun Sensor 4/1(S_B_hat), Sun Sensor 3/1(S_B_hat)
  Matrix Concatenate/1 -> S_S_m/1
  Inertial To Body/1 -> Eclipse Multiply/1
  Compare To Zero/1 -> Eclipse Multiply/2
  eclipse/1 -> Compare To Zero/1
  Sun Sensor 1/1(S_S1_m) -> Zero-Order Hold/1
  Sun Sensor 2/1(S_S2_m) -> Zero-Order Hold1/1
  Zero-Order Hold/1 -> Compare/1(Signal 1), Matrix Concatenate/1
  Zero-Order Hold1/1 -> Compare1/1(Signal 1), Matrix Concatenate/2
  Sun Sensor 1/2(S_S1) -> Compare/2(Signal 2)
  Compare/1(x) -> Sun Sensor Scooe 1/1
  Compare/2(y) -> Sun Sensor Scooe 1/2
  Compare/3(z) -> Sun Sensor Scooe 1/3
  Sun Sensor 3/1(S_S3_m) -> Zero-Order Hold2/1
  Sun Sensor 4/1(S_S4_m) -> Zero-Order Hold3/1
  Zero-Order Hold2/1 -> Compare2/1(Signal 1), Matrix Concatenate/3
  Zero-Order Hold3/1 -> Compare3/1(Signal 1), Matrix Concatenate/4
  Compare1/2(y) -> Sun Sensor Scooe 2/2
  Compare1/1(x) -> Sun Sensor Scooe 2/1
  Compare1/3(z) -> Sun Sensor Scooe 2/3
  Sun Sensor 2/2(S_S2) -> Compare1/2(Signal 2)
  Compare2/2(y) -> Sun Sensor Scooe 3/2
  Compare2/1(x) -> Sun Sensor Scooe 3/1
  Compare2/3(z) -> Sun Sensor Scooe 3/3
  Sun Sensor 3/2(S_S3) -> Compare2/2(Signal 2)
  Compare3/2(y) -> Sun Sensor Scooe 4/2
  Compare3/1(x) -> Sun Sensor Scooe 4/1
  Compare3/3(z) -> Sun Sensor Scooe 4/3
  Sun Sensor 4/2(S_S4) -> Compare3/2(Signal 2)

== system satellite_attitude_estimation_ekf_bst_model/Sensors/Gyro Sensor/Compare ==
  true : Inport
  real : Inport  Port=2
  Demux : Demux  Outputs=3
  Demux1 : Demux  Outputs=3
  Mux : Mux  Inputs=2
  Mux1 : Mux  Inputs=2
  Mux2 : Mux  Inputs=2
  x : Outport
  y : Outport  Port=2
  z : Outport  Port=3
  wires:
  Mux1/1 -> y/1
  Mux2/1 -> z/1
  true/1 -> Demux/1
  real/1 -> Demux1/1
  Mux/1 -> x/1
  Demux1/3 -> Mux2/2
  Demux1/2 -> Mux1/2
  Demux/3 -> Mux2/1
  Demux/1 -> Mux/1
  Demux/2 -> Mux1/1
  Demux1/1 -> Mux/2

== system satellite_attitude_estimation_ekf_bst_model/Sensors/Magnetometer/Compare ==
  true : Inport
  real : Inport  Port=2
  Demux : Demux  Outputs=3
  Demux1 : Demux  Outputs=3
  Mux : Mux  Inputs=2
  Mux1 : Mux  Inputs=2
  Mux2 : Mux  Inputs=2
  x : Outport
  y : Outport  Port=2
  z : Outport  Port=3
  wires:
  Mux1/1 -> y/1
  Mux2/1 -> z/1
  true/1 -> Demux/1
  real/1 -> Demux1/1
  Mux/1 -> x/1
  Demux1/3 -> Mux2/2
  Demux1/2 -> Mux1/2
  Demux/3 -> Mux2/1
  Demux/1 -> Mux/1
  Demux/2 -> Mux1/1
  Demux1/1 -> Mux/2

== system satellite_attitude_estimation_ekf_bst_model/Sensors/Sun Sensor/Compare ==
  Signal 1 : Inport
  Signal 2 : Inport  Port=2
  Demux3 : Demux  Outputs=3
  Demux4 : Demux  Outputs=3
  Mux : Mux  Inputs=2
  Mux1 : Mux  Inputs=2
  Mux2 : Mux  Inputs=2
  x : Outport
  y : Outport  Port=2
  z : Outport  Port=3
  wires:
  Demux3/3 -> Mux2/2
  Demux3/2 -> Mux1/2
  Demux4/2 -> Mux1/1
  Demux3/1 -> Mux/2
  Mux/1 -> x/1
  Mux2/1 -> z/1
  Demux4/1 -> Mux/1
  Mux1/1 -> y/1
  Demux4/3 -> Mux2/1
  Signal 2/1 -> Demux3/1
  Signal 1/1 -> Demux4/1

== system satellite_attitude_estimation_ekf_bst_model/Sensors/Sun Sensor/Compare1 ==
  Signal 1 : Inport
  Signal 2 : Inport  Port=2
  Demux3 : Demux  Outputs=3
  Demux4 : Demux  Outputs=3
  Mux : Mux  Inputs=2
  Mux1 : Mux  Inputs=2
  Mux2 : Mux  Inputs=2
  x : Outport
  y : Outport  Port=2
  z : Outport  Port=3
  wires:
  Demux3/3 -> Mux2/2
  Demux3/2 -> Mux1/2
  Demux4/2 -> Mux1/1
  Demux3/1 -> Mux/2
  Mux/1 -> x/1
  Mux2/1 -> z/1
  Demux4/1 -> Mux/1
  Mux1/1 -> y/1
  Demux4/3 -> Mux2/1
  Signal 2/1 -> Demux3/1
  Signal 1/1 -> Demux4/1

== system satellite_attitude_estimation_ekf_bst_model/Sensors/Sun Sensor/Compare2 ==
  Signal 1 : Inport
  Signal 2 : Inport  Port=2
  Demux3 : Demux  Outputs=3
  Demux4 : Demux  Outputs=3
  Mux : Mux  Inputs=2
  Mux1 : Mux  Inputs=2
  Mux2 : Mux  Inputs=2
  x : Outport
  y : Outport  Port=2
  z : Outport  Port=3
  wires:
  Demux3/3 -> Mux2/2
  Demux3/2 -> Mux1/2
  Demux4/2 -> Mux1/1
  Demux3/1 -> Mux/2
  Mux/1 -> x/1
  Mux2/1 -> z/1
  Demux4/1 -> Mux/1
  Mux1/1 -> y/1
  Demux4/3 -> Mux2/1
  Signal 2/1 -> Demux3/1
  Signal 1/1 -> Demux4/1

== system satellite_attitude_estimation_ekf_bst_model/Sensors/Sun Sensor/Compare3 ==
  Signal 1 : Inport
  Signal 2 : Inport  Port=2
  Demux3 : Demux  Outputs=3
  Demux4 : Demux  Outputs=3
  Mux : Mux  Inputs=2
  Mux1 : Mux  Inputs=2
  Mux2 : Mux  Inputs=2
  x : Outport
  y : Outport  Port=2
  z : Outport  Port=3
  wires:
  Demux3/3 -> Mux2/2
  Demux3/2 -> Mux1/2
  Demux4/2 -> Mux1/1
  Demux3/1 -> Mux/2
  Mux/1 -> x/1
  Mux2/1 -> z/1
  Demux4/1 -> Mux/1
  Mux1/1 -> y/1
  Demux4/3 -> Mux2/1
  Signal 2/1 -> Demux3/1
  Signal 1/1 -> Demux4/1

== system satellite_attitude_estimation_ekf_bst_model/Sensors/Sun Sensor/Sun Sensor 1 ==
  S_B_hat : Inport
  Compare To Constant : simulink/Logic and Bit Operations/Compare To Constant  relop=<  const=-cos(FOV/180*pi)  OutDataTypeStr=boolean
  Demux1 : Demux  Outputs=3
  Mux : Mux  Inputs=3
  Product1 : Product
  R_S1_B*(u) : Gain  Gain=R_S1_B  Multiplication=Matrix(K*u)
  SS Noise : RandomNumber  Variance=(sigSS*pi/180)^2  SampleTime=dt_ss
  Sum : Sum  Inputs=++|
  S_S1_m : Outport
  S_S1 : Outport  Port=2
  wires:
  S_B_hat/1 -> R_S1_B*(u)/1
  Demux1/2 -> Mux/2
  Demux1/3 -> Compare To Constant/1, Mux/3
  Demux1/1 -> Mux/1
  Compare To Constant/1 -> Product1/2
  Product1/1 -> S_S1_m/1
  Sum/1 -> Product1/1
  Mux/1 -> Sum/2
  SS Noise/1 -> Sum/1
  R_S1_B*(u)/1 -> S_S1/1, Demux1/1

== system satellite_attitude_estimation_ekf_bst_model/Sensors/Sun Sensor/Sun Sensor 2 ==
  S_B_hat : Inport
  Compare To Constant1 : simulink/Logic and Bit Operations/Compare To Constant  relop=<  const=-cos(FOV/180*pi)  OutDataTypeStr=boolean
  Demux2 : Demux  Outputs=3
  Mux1 : Mux  Inputs=3
  Product : Product
  R_S2_B*(u) : Gain  Gain=R_S2_B  Multiplication=Matrix(K*u)
  SS Noise : RandomNumber  Variance=(sigSS*pi/180)^2  SampleTime=dt_ss
  Sum : Sum  Inputs=++|
  S_S2_m : Outport
  S_S2 : Outport  Port=2
  wires:
  Product/1 -> S_S2_m/1
  R_S2_B*(u)/1 -> S_S2/1, Demux2/1
  Demux2/1 -> Mux1/1
  Demux2/2 -> Mux1/2
  Demux2/3 -> Compare To Constant1/1, Mux1/3
  Compare To Constant1/1 -> Product/2
  S_B_hat/1 -> R_S2_B*(u)/1
  Sum/1 -> Product/1
  SS Noise/1 -> Sum/1
  Mux1/1 -> Sum/2

== system satellite_attitude_estimation_ekf_bst_model/Sensors/Sun Sensor/Sun Sensor 3 ==
  S_B_hat : Inport
  Compare To Constant1 : simulink/Logic and Bit Operations/Compare To Constant  relop=<  const=-cos(FOV/180*pi)  OutDataTypeStr=boolean
  Demux2 : Demux  Outputs=3
  Mux1 : Mux  Inputs=3
  Product : Product
  R_S3_B*(u) : Gain  Gain=R_S3_B  Multiplication=Matrix(K*u)
  SS Noise : RandomNumber  Variance=(sigSS*pi/180)^2  SampleTime=dt_ss
  Sum : Sum  Inputs=++|
  S_S3_m : Outport
  S_S3 : Outport  Port=2
  wires:
  Product/1 -> S_S3_m/1
  R_S3_B*(u)/1 -> S_S3/1, Demux2/1
  Demux2/1 -> Mux1/1
  Demux2/2 -> Mux1/2
  Demux2/3 -> Compare To Constant1/1, Mux1/3
  Compare To Constant1/1 -> Product/2
  S_B_hat/1 -> R_S3_B*(u)/1
  Sum/1 -> Product/1
  SS Noise/1 -> Sum/1
  Mux1/1 -> Sum/2

== system satellite_attitude_estimation_ekf_bst_model/Sensors/Sun Sensor/Sun Sensor 4 ==
  S_B_hat : Inport
  Compare To Constant1 : simulink/Logic and Bit Operations/Compare To Constant  relop=<  const=-cos(FOV/180*pi)  OutDataTypeStr=boolean
  Demux2 : Demux  Outputs=3
  Mux1 : Mux  Inputs=3
  Product : Product
  R_S4_B*(u) : Gain  Gain=R_S4_B  Multiplication=Matrix(K*u)
  SS Noise : RandomNumber  Variance=(sigSS*pi/180)^2  SampleTime=dt_ss
  Sum : Sum  Inputs=++|
  S_S4_m : Outport
  S_S4 : Outport  Port=2
  wires:
  Product/1 -> S_S4_m/1
  R_S4_B*(u)/1 -> S_S4/1, Demux2/1
  Demux2/1 -> Mux1/1
  Demux2/2 -> Mux1/2
  Demux2/3 -> Compare To Constant1/1, Mux1/3
  Compare To Constant1/1 -> Product/2
  S_B_hat/1 -> R_S4_B*(u)/1
  Sum/1 -> Product/1
  SS Noise/1 -> Sum/1
  Mux1/1 -> Sum/2
